simulink model "batterySimulation"  (R2023b)
settings: Solver=VariableStepAuto  StartTime=0.0  StopTime=Sim_time  RelTol=1e-3
values from neighbouring files (symbols this model uses):
  Cn = 2.3*3600    (= 8280)    [ProjectBatteryRun.m]
  I = 2.3    [ProjectBatteryRun.m]
  OCV = Data(:,2)    [ProjectBatteryRun.m]
  R_Charge = Data(:,3)    [ProjectBatteryRun.m]
  R_Discharge = Data(:,4)    [ProjectBatteryRun.m]
  SOC = Data(:,1)    [ProjectBatteryRun.m]
settings Model: Creator=brlop  LastModifiedBy=brlop

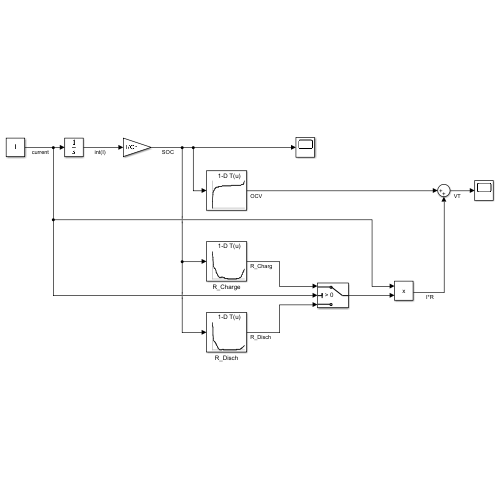
[thumbnail: Simulink's stored preview of the top-level diagram]
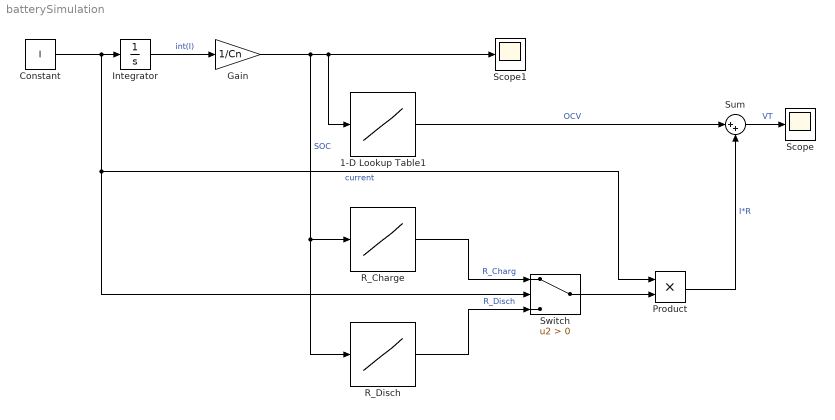
== system batterySimulation ==
  1-D Lookup Table1 : Lookup_n-D  NumberOfTableDimensions=1  BreakpointsForDimension1=SOC  Table=OCV  InternalRulePriority=Speed  RndMeth=Simplest
  Constant : Constant  Value=I
  Gain : Gain  Gain=1/Cn
  Integrator : Integrator
  Product : Product
  R_Charge : Lookup_n-D  NumberOfTableDimensions=1  BreakpointsForDimension1=SOC  Table=R_Charge  InternalRulePriority=Speed  RndMeth=Simplest
  R_Disch : Lookup_n-D  NumberOfTableDimensions=1  BreakpointsForDimension1=SOC  Table=R_Discharge  InternalRulePriority=Speed  RndMeth=Simplest
  Scope : Scope
  Scope1 : Scope
  Sum : Sum  Inputs=|++
  Switch : Switch  Criteria=u2 > Threshold  SaturateOnIntegerOverflow=off  InputSameDT=off
  wires:
  Constant/1 -> Product/1, Switch/2, Integrator/1  "current"
  Integrator/1 -> Gain/1  "int(I)"
  Gain/1 -> R_Disch/1, R_Charge/1, Scope1/1, 1-D Lookup Table1/1  "SOC"
  1-D Lookup Table1/1 -> Sum/1  "OCV"
  Product/1 -> Sum/2  "I*R"
  Sum/1 -> Scope/1  "VT"
  R_Charge/1 -> Switch/1  "R_Charg"
  R_Disch/1 -> Switch/3  "R_Disch"
  Switch/1 -> Product/2
